simulink model "DCservoclean"  (R2016a)
settings: Solver=VariableStepAuto  StartTime=0.0  StopTime=10.0  MaxStep=.01  RelTol=1e-3
settings Model: Creator=jordan  LastModifiedBy=jordan
settings DataIOCC: SaveOutput=off  SaveTime=off

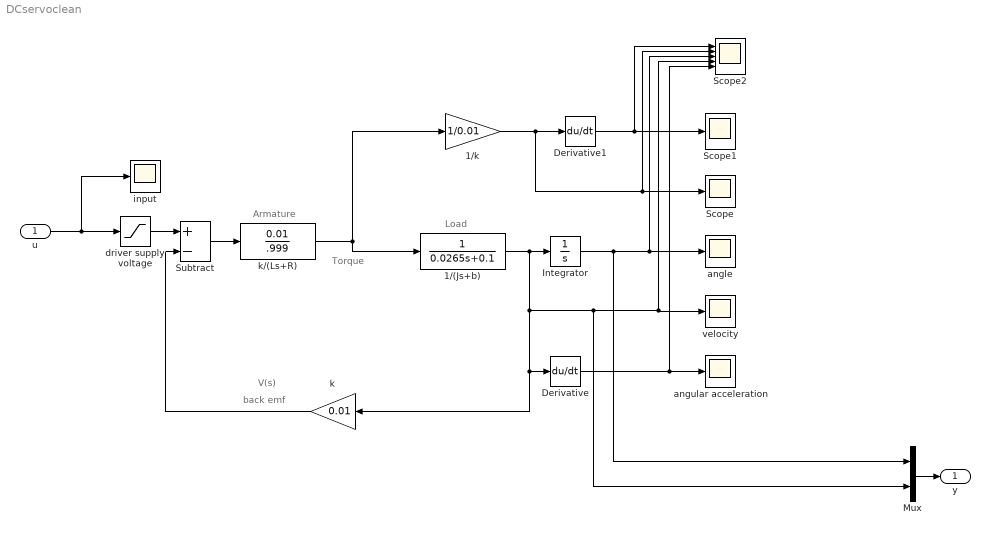
== system DCservoclean ==
  note: back emf
  note: Armature
  note: Torque
  note: Load
  note: V(s)
  u : Inport  OutDataTypeStr=double  PortDimensions=1  SampleTime=0
  1/(Js+b) : TransferFcn  Denominator=[0.0265 0.1]
  1/k : Gain  Gain=1/0.01
  Derivative : Derivative
  Derivative1 : Derivative
  Integrator : Integrator
  Mux : Mux  Inputs=2
  Scope : Scope
  Scope1 : Scope
  Scope2 : Scope  NumInputPorts=5
  Subtract : Sum  Inputs=+-
  angle : Scope
  angular acceleration : Scope
  driver supply voltage : Saturate  UpperLimit=48  LowerLimit=-48
  input : Scope
  k : Gain  Gain=0.01
  k/(Ls+R) : TransferFcn  Numerator=[0.01]  Denominator=[0 .999]
  velocity : Scope
  y : Outport  OutDataTypeStr=double  PortDimensions=2  SampleTime=0
  wires:
  1/(Js+b)/1 -> k/1, Derivative/1, Mux/2, Scope2/4, velocity/1, Integrator/1
  k/1 -> Subtract/2
  Subtract/1 -> k/(Ls+R)/1
  Derivative/1 -> Scope2/5, angular acceleration/1
  1/k/1 -> Derivative1/1, Scope/1, Scope2/2
  Derivative1/1 -> Scope2/1, Scope1/1
  Mux/1 -> y/1
  driver supply voltage/1 -> Subtract/1
  Integrator/1 -> Mux/1, Scope2/3, angle/1
  u/1 -> driver supply voltage/1, input/1
  k/(Ls+R)/1 -> 1/(Js+b)/1, 1/k/1
